simulink model "control_model_case_1_2"  (R2018a)
settings: Solver=VariableStepAuto  StartTime=0.0  StopTime=35  RelTol=1e-3
undefined symbols (not defined in the file): sigbuilder_block
libraries: fuzblock x3
settings Model: Creator=siati  LastModifiedBy=siati

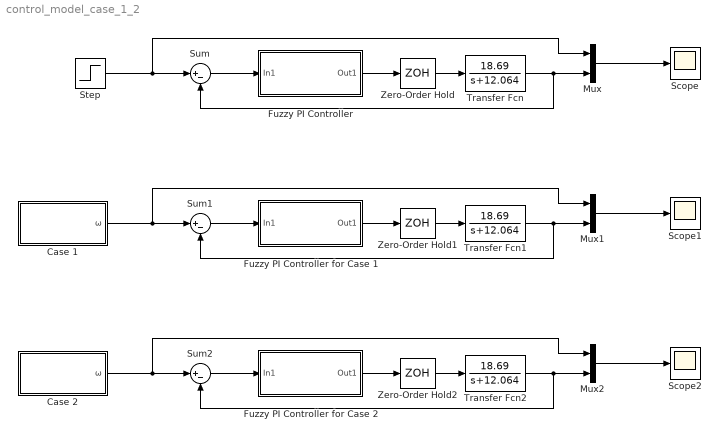
== system control_model_case_1_2 ==
  Case 1 : Subsystem  Tag=STV Subsys  LoadFcn=sigbuilder_block('load');  StartFcn=sigbuilder_block('start');  StopFcn=sigbuilder_block('stop');  ClipboardFcn=sigbuilder_block('clipboard');  mask(Sigbuilder block){tuvar=[0:10]}
      mask help: Simulink:masks:SigbuilderBlock_MD
      mask init:
      | if ~strcmp(get_param(bdroot(gcbh),'SimulationStatus'),'stopped') tuvar = sigbuilder_block('maskInit'); end
      settings: CopyFcn=sigbuilder_block('copy');  DeleteFcn=sigbuilder_block('delete');  ModelCloseFcn=sigbuilder_block('modelClose');  PreSaveFcn=sigbuilder_block('preSave');  PauseFcn=sigbuilder_block('pause');  ContinueFcn=sigbuilder_block('continue');  NameChangeFcn=sigbuilder_block('namechange');  OpenFcn=sigbuilder_block('open',[396.75 112.5 550.5 399.75 ]);  CloseFcn=sigbuilder_block('close');
      mask Display: plot(0, 0, 100, 100,[2, 2, 32, 32, 2], [68, 8, 8, 68, 68],[32, 2], [38, 38], [32, 19, 2],[53, 60, 44], [32, 17, 17, 2],[16, 16, 31, 31]);txt = getActiveGroup(gcbh);text(2, 100, txt,'verticalAlignment', 'top');
  Case 2 : Subsystem  Tag=STV Subsys  LoadFcn=sigbuilder_block('load');  StartFcn=sigbuilder_block('start');  StopFcn=sigbuilder_block('stop');  ClipboardFcn=sigbuilder_block('clipboard');  mask(Sigbuilder block){tuvar=[0:10]}
      mask help: Simulink:masks:SigbuilderBlock_MD
      mask init:
      | if ~strcmp(get_param(bdroot(gcbh),'SimulationStatus'),'stopped') tuvar = sigbuilder_block('maskInit'); end
      settings: CopyFcn=sigbuilder_block('copy');  DeleteFcn=sigbuilder_block('delete');  ModelCloseFcn=sigbuilder_block('modelClose');  PreSaveFcn=sigbuilder_block('preSave');  PauseFcn=sigbuilder_block('pause');  ContinueFcn=sigbuilder_block('continue');  NameChangeFcn=sigbuilder_block('namechange');  OpenFcn=sigbuilder_block('open',[330.75 132 550.5 399.75 ]);  CloseFcn=sigbuilder_block('close');
      mask Display: plot(0, 0, 100, 100,[2, 2, 32, 32, 2], [68, 8, 8, 68, 68],[32, 2], [38, 38], [32, 19, 2],[53, 60, 44], [32, 17, 17, 2],[16, 16, 31, 31]);txt = getActiveGroup(gcbh);text(2, 100, txt,'verticalAlignment', 'top');
  Fuzzy PI Controller : Subsystem
  Fuzzy PI Controller for Case 1 : Subsystem
  Fuzzy PI Controller for Case 2 : Subsystem
  Mux : Mux  Inputs=2
  Mux1 : Mux  Inputs=2
  Mux2 : Mux  Inputs=2
  Scope : Scope
  Scope1 : Scope
  Scope2 : Scope
  Step : Step  After=150  SampleTime=0.01
  Sum : Sum  Inputs=|+-
  Sum1 : Sum  Inputs=|+-
  Sum2 : Sum  Inputs=|+-
  Transfer Fcn : TransferFcn  Numerator=[18.69]  Denominator=[1 12.064]
  Transfer Fcn1 : TransferFcn  Numerator=[18.69]  Denominator=[1 12.064]
  Transfer Fcn2 : TransferFcn  Numerator=[18.69]  Denominator=[1 12.064]
  Zero-Order Hold : ZeroOrderHold  SampleTime=-1
  Zero-Order Hold1 : ZeroOrderHold  SampleTime=-1
  Zero-Order Hold2 : ZeroOrderHold  SampleTime=-1
  wires:
  Step/1 -> Mux/1, Sum/1
  Sum/1 -> Fuzzy PI Controller/1(In1)
  Fuzzy PI Controller/1(Out1) -> Zero-Order Hold/1
  Zero-Order Hold/1 -> Transfer Fcn/1
  Transfer Fcn/1 -> Sum/2, Mux/2
  Mux/1 -> Scope/1
  Case 1/1(ω) -> Mux1/1, Sum1/1
  Fuzzy PI Controller for Case 1/1(Out1) -> Zero-Order Hold1/1
  Transfer Fcn1/1 -> Sum1/2, Mux1/2
  Mux1/1 -> Scope1/1
  Zero-Order Hold1/1 -> Transfer Fcn1/1
  Sum1/1 -> Fuzzy PI Controller for Case 1/1(In1)
  Sum2/1 -> Fuzzy PI Controller for Case 2/1(In1)
  Zero-Order Hold2/1 -> Transfer Fcn2/1
  Transfer Fcn2/1 -> Sum2/2, Mux2/2
  Mux2/1 -> Scope2/1
  Fuzzy PI Controller for Case 2/1(Out1) -> Zero-Order Hold2/1
  Case 2/1(ω) -> Mux2/1, Sum2/1

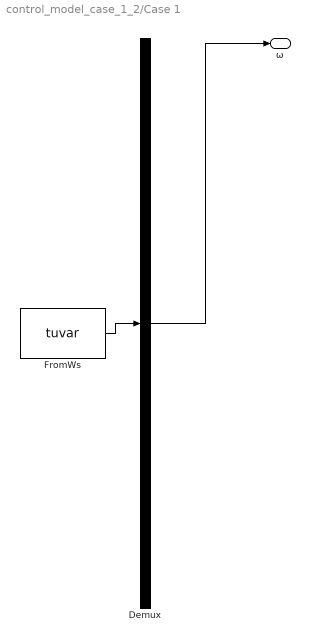
== system control_model_case_1_2/Case 1 ==
  Demux : Demux  Tag=STV Demux  Outputs=1
  FromWs : FromWorkspace  Tag=STV FromWs  VariableName=tuvar  SampleTime=0
      SigBuilderData=|
      | common.afterFinalStr = 'Extrapolate'
      | common.sampleTime = 0
      | dataSet.timeRange = [0 30]
      | dataSet.name = 'Group 1'
      | sbobj.Groups.Name = 'Group 1'
      | sbobj.Groups.Signals.Name = 'ω'
      | sbobj.Groups.Signals.XData = [0 10 10 20 20 30]
      | sbobj.Groups.Signals.YData = [150 150 100 100 150 150]
      | sbobj.Groups.TimeRange = [0 30]
  ω : Outport  Tag=STV Outport
  wires:
  Demux/1 -> ω/1
  FromWs/1 -> Demux/1

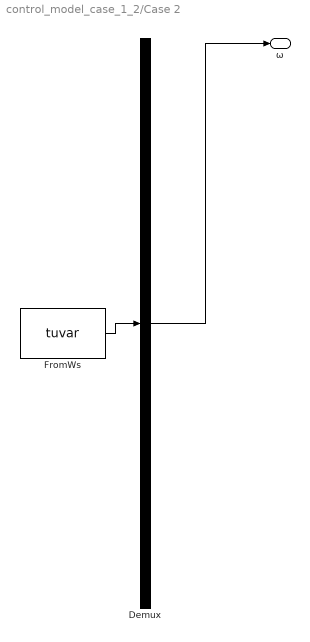
== system control_model_case_1_2/Case 2 ==
  Demux : Demux  Tag=STV Demux  Outputs=1
  FromWs : FromWorkspace  Tag=STV FromWs  VariableName=tuvar  SampleTime=0
      SigBuilderData=|
      | common.afterFinalStr = 'Extrapolate'
      | common.sampleTime = 0
      | dataSet.timeRange = [0 30]
      | dataSet.name = 'Group 1'
      | sbobj.Groups.Name = 'Group 1'
      | sbobj.Groups.Signals.Name = 'ω'
      | sbobj.Groups.Signals.XData = [0 10 20 30]
      | sbobj.Groups.Signals.YData = [0 150 150 0]
      | sbobj.Groups.TimeRange = [0 30]
  ω : Outport  Tag=STV Outport
  wires:
  Demux/1 -> ω/1
  FromWs/1 -> Demux/1

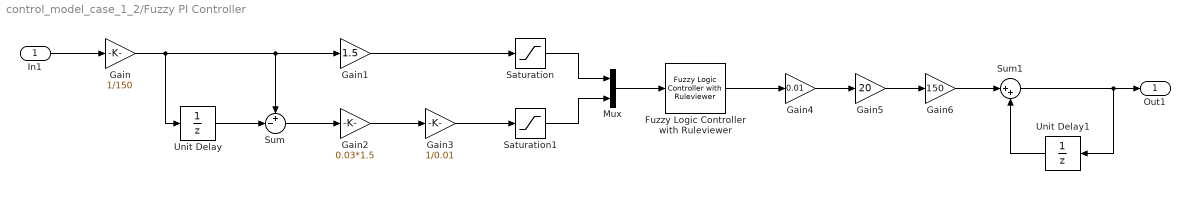
== system control_model_case_1_2/Fuzzy PI Controller ==
  In1 : Inport
  Fuzzy Logic Controller with Ruleviewer : fuzblock/Fuzzy Logic  Controller  with Ruleviewer  fismatrix=FLC  Ts=1
  Gain : Gain  Gain=1/150
  Gain1 : Gain  Gain=1.5
  Gain2 : Gain  Gain=0.03*1.5
  Gain3 : Gain  Gain=1/0.01
  Gain4 : Gain  Gain=0.01
  Gain5 : Gain  Gain=20
  Gain6 : Gain  Gain=150
  Mux : Mux  Inputs=2
  Saturation : Saturate
  Saturation1 : Saturate
  Sum : Sum  Inputs=+-|
  Sum1 : Sum  Inputs=|++
  Unit Delay : UnitDelay  SampleTime=-1
  Unit Delay1 : UnitDelay  SampleTime=-1
  Out1 : Outport
  wires:
  Gain4/1 -> Gain5/1
  Gain5/1 -> Gain6/1
  In1/1 -> Gain/1
  Gain/1 -> Sum/1, Gain1/1, Unit Delay/1
  Unit Delay/1 -> Sum/2
  Sum/1 -> Gain2/1
  Gain2/1 -> Gain3/1
  Gain1/1 -> Saturation/1
  Gain3/1 -> Saturation1/1
  Saturation/1 -> Mux/1
  Saturation1/1 -> Mux/2
  Mux/1 -> Fuzzy Logic Controller with Ruleviewer/1
  Gain6/1 -> Sum1/1
  Unit Delay1/1 -> Sum1/2
  Sum1/1 -> Out1/1, Unit Delay1/1
  Fuzzy Logic Controller with Ruleviewer/1 -> Gain4/1

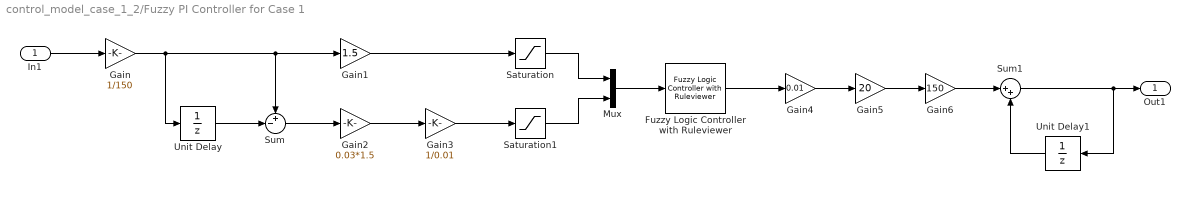
== system control_model_case_1_2/Fuzzy PI Controller for Case 1 ==
  In1 : Inport
  Fuzzy Logic Controller with Ruleviewer : fuzblock/Fuzzy Logic  Controller  with Ruleviewer  fismatrix=FLC  Ts=1
  Gain : Gain  Gain=1/150
  Gain1 : Gain  Gain=1.5
  Gain2 : Gain  Gain=0.03*1.5
  Gain3 : Gain  Gain=1/0.01
  Gain4 : Gain  Gain=0.01
  Gain5 : Gain  Gain=20
  Gain6 : Gain  Gain=150
  Mux : Mux  Inputs=2
  Saturation : Saturate
  Saturation1 : Saturate
  Sum : Sum  Inputs=+-|
  Sum1 : Sum  Inputs=|++
  Unit Delay : UnitDelay  SampleTime=-1
  Unit Delay1 : UnitDelay  SampleTime=-1
  Out1 : Outport
  wires:
  Gain4/1 -> Gain5/1
  Gain5/1 -> Gain6/1
  In1/1 -> Gain/1
  Gain/1 -> Sum/1, Gain1/1, Unit Delay/1
  Unit Delay/1 -> Sum/2
  Sum/1 -> Gain2/1
  Gain2/1 -> Gain3/1
  Gain1/1 -> Saturation/1
  Gain3/1 -> Saturation1/1
  Saturation/1 -> Mux/1
  Saturation1/1 -> Mux/2
  Mux/1 -> Fuzzy Logic Controller with Ruleviewer/1
  Gain6/1 -> Sum1/1
  Unit Delay1/1 -> Sum1/2
  Sum1/1 -> Out1/1, Unit Delay1/1
  Fuzzy Logic Controller with Ruleviewer/1 -> Gain4/1

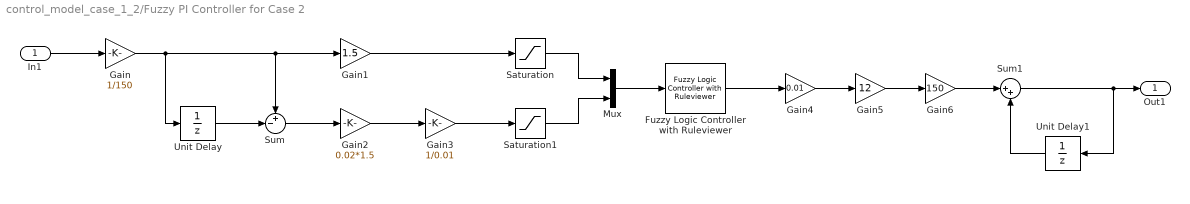
== system control_model_case_1_2/Fuzzy PI Controller for Case 2 ==
  In1 : Inport
  Fuzzy Logic Controller with Ruleviewer : fuzblock/Fuzzy Logic  Controller  with Ruleviewer  fismatrix=FLC  Ts=1
  Gain : Gain  Gain=1/150
  Gain1 : Gain  Gain=1.5
  Gain2 : Gain  Gain=0.02*1.5
  Gain3 : Gain  Gain=1/0.01
  Gain4 : Gain  Gain=0.01
  Gain5 : Gain  Gain=12
  Gain6 : Gain  Gain=150
  Mux : Mux  Inputs=2
  Saturation : Saturate
  Saturation1 : Saturate
  Sum : Sum  Inputs=+-|
  Sum1 : Sum  Inputs=|++
  Unit Delay : UnitDelay  SampleTime=-1
  Unit Delay1 : UnitDelay  SampleTime=-1
  Out1 : Outport
  wires:
  Gain4/1 -> Gain5/1
  Gain5/1 -> Gain6/1
  In1/1 -> Gain/1
  Gain/1 -> Sum/1, Gain1/1, Unit Delay/1
  Unit Delay/1 -> Sum/2
  Sum/1 -> Gain2/1
  Gain2/1 -> Gain3/1
  Gain1/1 -> Saturation/1
  Gain3/1 -> Saturation1/1
  Saturation/1 -> Mux/1
  Saturation1/1 -> Mux/2
  Mux/1 -> Fuzzy Logic Controller with Ruleviewer/1
  Gain6/1 -> Sum1/1
  Unit Delay1/1 -> Sum1/2
  Sum1/1 -> Out1/1, Unit Delay1/1
  Fuzzy Logic Controller with Ruleviewer/1 -> Gain4/1
